simulink model "ADHW2p3"  (R2022a)
settings: Solver=VariableStepAuto  StartTime=0.0  StopTime=10.0  RelTol=1e-3
settings Model: Creator=izacu  LastModifiedBy=izacu

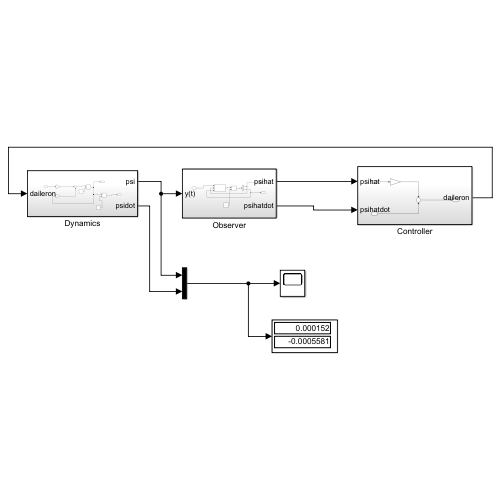
[thumbnail: Simulink's stored preview of the top-level diagram]
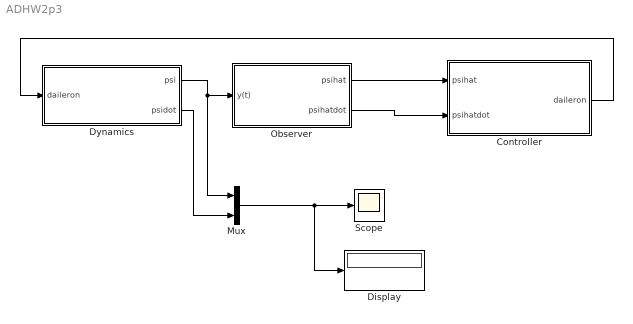
== system ADHW2p3 ==
  Controller : Subsystem
  Display : Display
  Dynamics : Subsystem
  Mux : Mux  Inputs=2
  Observer : Subsystem
  Scope : Scope
  wires:
  Controller/1(daileron) -> Dynamics/1(daileron)
  Dynamics/1(psi) -> Mux/1, Observer/1(y(t))
  Observer/1(psihat) -> Controller/1(psihat)
  Observer/2(psihatdot) -> Controller/2(psihatdot)
  Mux/1 -> Display/1, Scope/1
  Dynamics/2(psidot) -> Mux/2

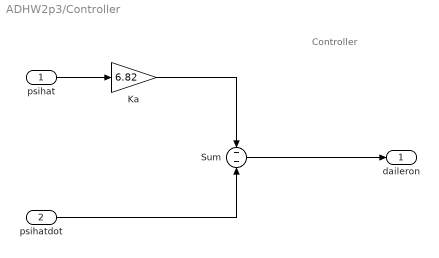
== system ADHW2p3/Controller ==
  note: Controller
  psihat : Inport
  psihatdot : Inport  Port=2
  Ka : Gain  Gain=6.82
  Sum : Sum  Inputs=--
  daileron : Outport
  wires:
  psihat/1 -> Ka/1
  Sum/1 -> daileron/1
  Ka/1 -> Sum/1
  psihatdot/1 -> Sum/2

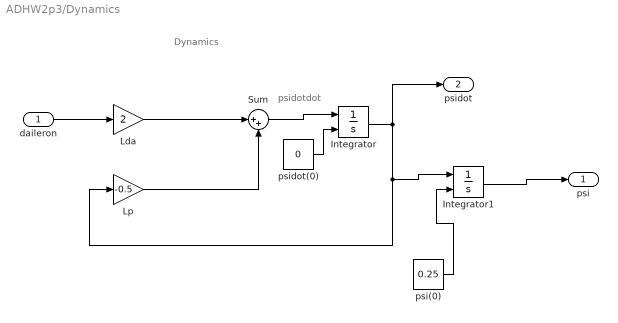
== system ADHW2p3/Dynamics ==
  note: Dynamics
  note: psidotdot
  daileron : Inport
  Integrator : Integrator  InitialConditionSource=external
  Integrator1 : Integrator  InitialConditionSource=external
  Lda : Gain  Gain=2
  Lp : Gain  Gain=-0.5
  Sum : Sum  Inputs=|++
  psi(0) : Constant  Value=0.25
  psidot(0) : Constant  Value=0
  psi : Outport
  psidot : Outport  Port=2
  wires:
  Lda/1 -> Sum/1
  Lp/1 -> Sum/2
  Sum/1 -> Integrator/1
  daileron/1 -> Lda/1
  Integrator/1 -> Lp/1, Integrator1/1, psidot/1
  psidot(0)/1 -> Integrator/2
  Integrator1/1 -> psi/1
  psi(0)/1 -> Integrator1/2

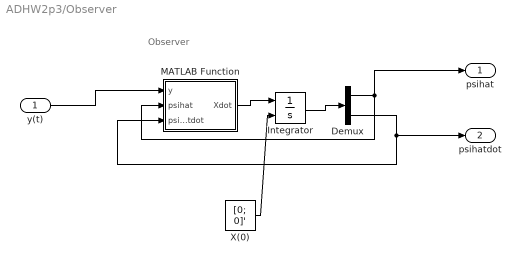
== system ADHW2p3/Observer ==
  note: Observer
  y(t) : Inport
  Demux : Demux  Outputs=2
  Integrator : Integrator  InitialConditionSource=external
  MATLAB Function : MATLAB Function  TreatAsAtomicUnit=on
  X(0) : Constant  Value=[0; 0]'
  psihat : Outport
  psihatdot : Outport  Port=2
  wires:
  MATLAB Function/1(Xdot) -> Integrator/1
  Integrator/1 -> Demux/1
  X(0)/1 -> Integrator/2
  Demux/1 -> psihat/1, MATLAB Function/2(psihat)
  Demux/2 -> psihatdot/1, MATLAB Function/3(psihatdot)
  y(t)/1 -> MATLAB Function/1(y)

== matlab function ADHW2p3/Observer/MATLAB Function ==
  data: y input; Xdot output; psihat input; psihatdot input
function Xdot = fcn(y,psihat,psihatdot)
X = [psihat; psihatdot];
A = [0 1; -6.82 -1];
L = [50; 50];

Xdot = A*X + L*(y - psihat);
